simulink model "solarmonitor"  (R2019b)
settings: Solver=FixedStepAuto  StartTime=0.0  StopTime=10.0  RelTol=1e-3  EnableMultiTasking=on
libraries: raspberrypilib x2
settings Model: SimulationMode=external  Creator=shogo  LastModifiedBy=shogo
settings SolverCC: PositivePriorityOrder=on
settings OptimizationCC: EnhancedBackFolding=on  PassReuseOutputArgsAs=Individual arguments  ZeroExternalMemoryAtStartup=off  ZeroInternalMemoryAtStartup=off  MaxStackSize=64  OptimizeBlockOrder=speed  DifferentSizesBufferReuse=on  OptimizationCustomize=off  EfficientTunableParamExpr=on
settings DebuggingCC: ParameterTunabilityLossMsg=error
settings HardwareCC: ProdBitPerPointer=32  ProdBitPerSizeT=32  ProdBitPerPtrDiffT=32  ProdLargestAtomicInteger=Long  ProdLargestAtomicFloat=Double  ProdWordSize=32  ProdLongLongMode=on  ProdHWDeviceType=ARM Compatible->ARM Cortex  UseEmbeddedCoderFeatures=off  UseSimulinkCoderFeatures=off
settings RTWCC: SystemTargetFile=ert.tlc  HardwareBoard=Raspberry Pi  TLCOptions="-aInlineSetEventsForThisBaseRateFcn=TLC_FALSE -aSuppressMultiTaskScheduler=TLC_FALSE  -aRateBasedStepFcn=0"  TemplateMakefile=ert_default_tmf  RTWVerbose=off  Toolchain=GNU GCC Raspberry Pi  BuildConfiguration=Faster Runs  IncludeHyperlinkInReport=on
settings CodeAppCC: ForceParamTrailComments=on  OperatorAnnotations=on  SimulinkDataObjDesc=on  SFDataObjDesc=on  MangleLength=10  InsertBlockDesc=on
settings ERTTargetCC: SupportNonInlinedSFcns=on  SupportVariableSizeSignals=on  ExtMode=on  ExtModeTransport=2  ExtModeStaticAlloc=on  ExtModeMexFile=ext_xcp  ExtModeMexArgs='192.168.11.21' 0 17725  ExtModeIntrfLevel=Level2 - Open  ERTSrcFileBannerTemplate=codertarget_code_template.cgt  ERTHdrFileBannerTemplate=codertarget_code_template.cgt  ERTDataSrcFileTemplate=codertarget_code_template.cgt  ERTDataHdrFileTemplate=codertarget_code_template.cgt

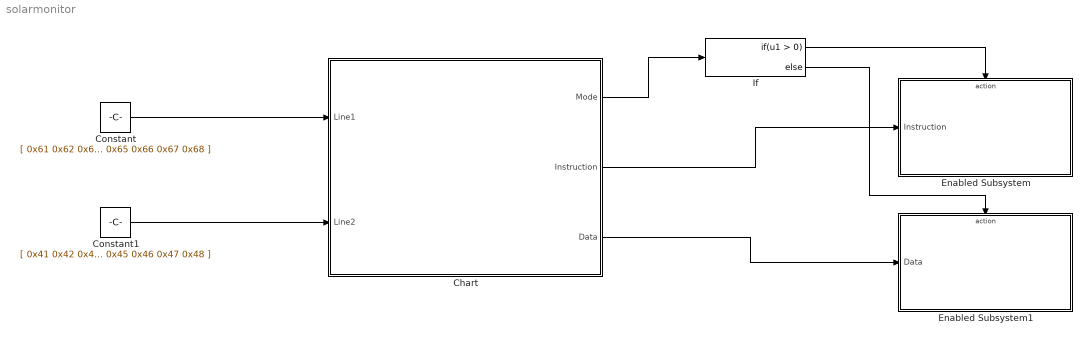
== system solarmonitor ==
  Chart : Stateflow chart  BlockKeywords=__PRM__SERIALIZED__DATA__:Stateflow Chart,Stateflow Diagram  TreatAsAtomicUnit=on
  Constant : Constant  Value=[ 0x61 0x62 0x63 0x64 0x65 0x66 0x67 0x68 ]
  Constant1 : Constant  Value=[ 0x41 0x42 0x43 0x44 0x45 0x46 0x47 0x48 ]
  Enabled Subsystem : Subsystem  TreatAsAtomicUnit=on
  Enabled Subsystem1 : Subsystem  TreatAsAtomicUnit=on
  If : If
  wires:
  Chart/3(Data) -> Enabled Subsystem1/1(Data)
  Chart/2(Instruction) -> Enabled Subsystem/1(Instruction)
  Chart/1(Mode) -> If/1
  If/1 -> Enabled Subsystem/Action
  If/2 -> Enabled Subsystem1/Action
  Constant/1 -> Chart/1(Line1)
  Constant1/1 -> Chart/2(Line2)

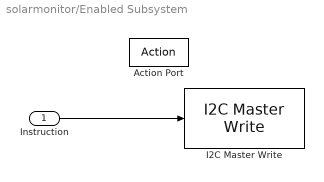
== system solarmonitor/Enabled Subsystem ==
  Instruction : Inport
  Action Port : ActionPort  ActionPortLabel=if(u1 > 0)
  I2C Master Write : raspberrypilib/I2C Master Write  BoardProperty=Pi 3 Model B  Mode=Master  SlaveAddress=0x3e  SlaveByteOrder=BigEndian  Direction=Transmitter  RegisterAddressMode=on  RegisterAddress=0x00  SlaveDataType=uint8  DataLength=1  NoAck=off  RepeatedStart=off  OutputStatus=off
      settings: SourceProductName=Simulink Support Package for Raspberry Pi Hardware  SourceProductBaseCode=RASPPI
  wires:
  Instruction/1 -> I2C Master Write/1

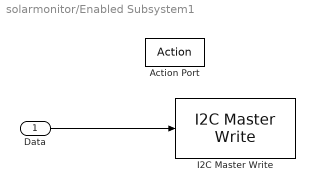
== system solarmonitor/Enabled Subsystem1 ==
  Data : Inport
  Action Port : ActionPort  ActionPortLabel=else
  I2C Master Write : raspberrypilib/I2C Master Write  BoardProperty=Pi 3 Model B  Mode=Master  SlaveAddress=0x3e  SlaveByteOrder=BigEndian  Direction=Transmitter  RegisterAddressMode=on  RegisterAddress=0x40  SlaveDataType=uint8  DataLength=1  NoAck=off  RepeatedStart=off  OutputStatus=off
      settings: SourceProductName=Simulink Support Package for Raspberry Pi Hardware  SourceProductBaseCode=RASPPI
  wires:
  Data/1 -> I2C Master Write/1

== stateflow chart solarmonitor/Chart ==
  state Display_1st_char_in_line1
    Mode = 0;
    idx = 1;
    Data = Line1(idx);
  state Initalization
    Mode = 1;
  state Function_set1
    Instruction = 0x38;
  state Display_line1
    Data = Line1(idx);
  state Function_set2
    Instruction = 0x39;
  state Internal_OSC_Freq
    Instruction = 0x14;
  state Move_to_line2
    Mode = 1;
    Instruction = 0xc0;
  state Contrast_set
    Instruction = 0x73;
  state PW_ICN_CNT_Ctrl
    Instruction = 0x56;
  state Display_1st_char_in_line2
    Mode = 0;
    idx = 1;
    Data = Line2(idx);
  state Follower_Ctrl
    Instruction = 0x6c
  state Display_line2
    Data = Line2(idx);
  state Function_set3
    Instruction = 0x38;
  state Display_On_Off_Ctrl
    Instruction = 0x0c;
  state Move_to_line1
    Mode = 1;
    Instruction = 0x80;
  state Clear_display
    Instruction = 0x01;
  (default) -> Initalization
  Move_to_line1 -> Display_1st_char_in_line1
  Initalization -> Function_set1
  Clear_display -> Display_1st_char_in_line1 : after(1,msec)
  Display_1st_char_in_line1 -> Display_line1 : {idx=idx+1;}
  Function_set1 -> Function_set2
  Display_line1 -> Display_line1 [order 1] : [idx<8]{idx=idx+1;}
  Function_set2 -> Internal_OSC_Freq
  Display_line1 -> Move_to_line2 [order 2]
  Internal_OSC_Freq -> Contrast_set
  Move_to_line2 -> Display_1st_char_in_line2
  Contrast_set -> PW_ICN_CNT_Ctrl
  PW_ICN_CNT_Ctrl -> Follower_Ctrl
  Display_1st_char_in_line2 -> Display_line2 : {idx=idx+1;}
  Follower_Ctrl -> Function_set3 : after(200,msec)
  Display_line2 -> Display_line2 [order 1] : [idx<8]{idx=idx+1;}
  Function_set3 -> Display_On_Off_Ctrl
  Display_line2 -> Move_to_line1 [order 2]
  Display_On_Off_Ctrl -> Clear_display
  data: Mode output; Instruction output; Data output; Line1 input; Line2 input
